simulink model "andbot1dot2_voltage_loop_frictioncompensation"  (R2015b)
settings: Solver=FixedStepAuto  StartTime=0.0  StopTime=simulation_time  FixedStep=0.04  RelTol=1e-3
values from neighbouring files (symbols this model uses):
  den_ff_Omega = [0 3.2393]    [andbot1dot2_MIMO_modeling_omega_loop.m]
  den_ff_Vel = [0 1.054]    [andbot1dot2_MIMO_modeling_vel_loop.m]
  den_Omega = [1 4.9887]    [andbot1dot2_MIMO_modeling.m]    (also in andbot1dot2_MIMO_modeling_omega_loop.m)
  den_Vel = [1 2.5006]    [andbot1dot2_MIMO_modeling.m]    (also in andbot1dot2_MIMO_modeling_vel_loop.m = [1 6.313])
  gain_anti_windup_Vel = 10    [andbot1dot2_MIMO_modeling_vel_loop.m]
  input_Omega = 1    [andbot1dot2_MIMO_modeling.m]
  input_Vel = 1    [andbot1dot2_MIMO_modeling.m]
  Ki_Omega = 0    [andbot1dot2_MIMO_modeling.m]    (also in andbot1dot2_MIMO_modeling_omega_loop.m = 5.8287)
  Ki_Vel = 1    [andbot1dot2_MIMO_modeling.m]    (also in andbot1dot2_MIMO_modeling_vel_loop.m = 21.3962)
  Kp_Omega = 1    [andbot1dot2_MIMO_modeling.m]    (also in andbot1dot2_MIMO_modeling_omega_loop.m = 4.4157)
  Kp_Vel = 1500    [andbot1dot2_MIMO_modeling.m]    (also in andbot1dot2_MIMO_modeling_vel_loop.m = 14.9624)
  num_ff_Omega = [0 4.99887]    [andbot1dot2_MIMO_modeling_omega_loop.m]
  num_ff_Vel = [0 6.313]    [andbot1dot2_MIMO_modeling_vel_loop.m]
  num_Omega = [0 3.2393]    [andbot1dot2_MIMO_modeling.m]    (also in andbot1dot2_MIMO_modeling_omega_loop.m)
  num_Vel = [0 0.261065]    [andbot1dot2_MIMO_modeling.m]    (also in andbot1dot2_MIMO_modeling_vel_loop.m = [0 1.054])
  Tsample = 0.04    [andbot1dot2_param.m]
  Vq_MAX = 1000    [andbot1dot2_param.m]
undefined symbols (not defined in the file or in its folder): ENCOutputMode, gain_anti_windup_Omega, PracLoopDelay, SetENCSample, Umax_Volt, Umin_Volt
libraries: cstblocks x4, realtime_pacer_lib x2, slctrlblks x1
settings Model: Creator=shangwei  LastModifiedBy=root

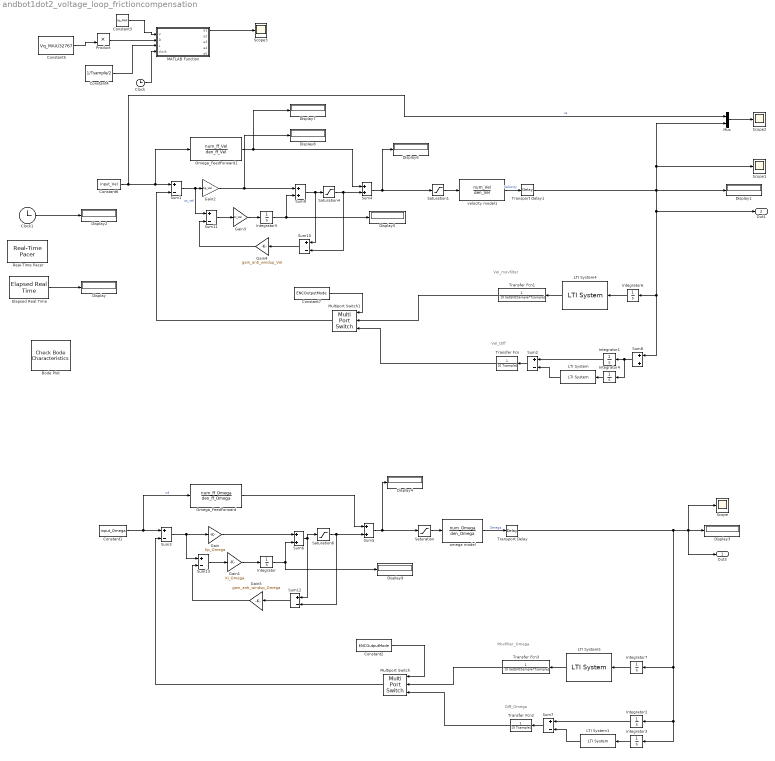
== system andbot1dot2_voltage_loop_frictioncompensation ==
  note: Vel_movfilter
  note: Diff_Omega
  note: Vel_Diff
  note: Movfilter_Omega
  Bode Plot : slctrlblks/Model Verification/Check Bode  Characteristics  InstantiateOnLoad=on  SaveOperatingPoints=off  LinearizationIOs={'/Sum1', 1, 'outin', 'on', '';'/Sum3', 1, 'outin', 'on', ''}  LinearizeAt=SnapshotTimes  SnapshotTimes=[0]  TriggerType=rising  SampleTime=auto  RateConversionMethod=zoh  PreWarpFreq=10  UseExactDelayModel=on  UseFullBlockNameLabels=off  UseBusSignalLabels=off  enabled=on  stopWhenAssertionFail=off  export=off  ViewDlgPos=[3023 418 520 393]  OpenViewOnLoad=off  LaunchViewOnOpen=on  FrequencyUnits=rad/s  MagnitudeUnits=dB  PhaseUnits=deg  TimeUnits=seconds  EnableUpperBound=off  UpperBoundFrequencies=[]  UpperBoundMagnitudes=[]  EnableLowerBound=off  LowerBoundFrequencies=[]  LowerBoundMagnitudes=[]
  Clock : Clock
  Clock1 : Clock
  Constant1 : Constant  Value=input_Omega  SampleTime=-1
  Constant2 : Constant  Value=ENCOutputMode  SampleTime=-1
  Constant3 : Constant  Value=Vq_MAX  SampleTime=-1
  Constant4 : Constant  Value=1/Tsample/2  SampleTime=-1
  Constant5 : Constant  Value=Vq_MAX/32767  SampleTime=-1
  Constant6 : Constant  Value=input_Vel  SampleTime=-1
  Constant7 : Constant  Value=ENCOutputMode  SampleTime=-1
  Display{,1..9} (10 alike) : Display
  Elapsed Real Time : realtime_pacer_lib/Elapsed Real Time
  Gain : Gain  Gain=Kp_Omega
  Gain1 : Gain  Gain=Ki_Omega
  Gain2 : Gain  Gain=Kp_Vel
  Gain3 : Gain  Gain=Ki_Vel
  Gain4 : Gain  Gain=gain_anti_windup_Vel
  Gain5 : Gain  Gain=gain_anti_windup_Omega
  Integrator{,1..7} (8 alike) : Integrator
  LTI System : cstblocks/LTI System  sys=time_delay_tf  IC=[]
  LTI System1 : cstblocks/LTI System  sys=time_delay_tf  IC=[]
  LTI System4 : cstblocks/LTI System  sys=(1 - exp(-SetENCSample*Tsample*tf('s'))) / (1 - exp(-Tsample*tf('s')))  IC=[]
  LTI System5 : cstblocks/LTI System  sys=(1 - exp(-SetENCSample*Tsample*tf('s'))) / (1 - exp(-Tsample*tf('s')))  IC=[]
  MATLAB Function : MATLAB Function  TreatAsAtomicUnit=on
  Multiport Switch : MultiPortSwitch  Inputs=2
  Multiport Switch1 : MultiPortSwitch  Inputs=2
  Mux : Mux  Inputs=2
  Omega_FeedForward : TransferFcn  Numerator=num_ff_Omega  Denominator=den_ff_Omega
  Omega_FeedForward1 : TransferFcn  Numerator=num_ff_Vel  Denominator=den_ff_Vel
  Product : Product
  Real-Time Pacer : realtime_pacer_lib/Real-Time Pacer  simTimePerRealTime=1
  Saturation{,1,4,6} (4 alike) : Saturate  UpperLimit=Umax_Volt  LowerLimit=Umin_Volt
  Scope{,1..3} (4 alike) : Scope
  Sum{1..3,7,10..13} (8 alike) : Sum  Inputs=+-
  Sum{4..6,8..9} (5 alike) : Sum
  Transfer Fcn : TransferFcn  Denominator=[0 Tsample]
  Transfer Fcn1 : TransferFcn  Denominator=[0 SetENCSample*Tsample]
  Transfer Fcn2 : TransferFcn  Denominator=[0 Tsample]
  Transfer Fcn3 : TransferFcn  Denominator=[0 SetENCSample*Tsample]
  Transport Delay : TransportDelay  DelayTime=PracLoopDelay
  Transport Delay1 : TransportDelay  DelayTime=PracLoopDelay
  omega model : TransferFcn  Numerator=num_Omega  Denominator=den_Omega
  velocity model1 : TransferFcn  Numerator=num_Vel  Denominator=den_Vel
  Out3 : Outport
  Out1 : Outport  Port=2
  wires:
  Sum3/1 -> Sum13/1, Gain/1
  Constant1/1 -> Sum3/1, Omega_FeedForward/1  "ud"
  Sum6/1 -> Saturation6/1, Sum12/1
  Sum1/1 -> Sum11/1, Gain2/1  "us_vel"
  velocity model1/1 -> Transport Delay1/1  "Velocity"
  Constant6/1 -> Mux/1, Sum1/1, Omega_FeedForward1/1  "us"
  omega model/1 -> Transport Delay/1  "Omega"
  Integrator3/1 -> LTI System1/1
  Integrator2/1 -> Sum7/1
  LTI System1/1 -> Sum7/2
  Sum7/1 -> Transfer Fcn2/1
  Sum2/1 -> Transfer Fcn/1
  Sum8/1 -> Integrator1/1, Integrator4/1
  Integrator1/1 -> Sum2/1
  LTI System/1 -> Sum2/2
  Integrator4/1 -> LTI System/1
  Constant3/1 -> MATLAB Function/1(V)
  MATLAB Function/1(a1) -> Scope3/1
  Product/1 -> MATLAB Function/2(D)
  Constant4/1 -> MATLAB Function/3(L)
  Clock/1 -> MATLAB Function/4(clock)
  Constant5/1 -> Product/2
  Multiport Switch/1 -> Sum3/2
  Transport Delay1/1 -> Display1/1, Scope1/1, Mux/2, Out1/1, Integrator6/1, Sum8/1
  Gain1/1 -> Integrator/1
  Gain/1 -> Sum6/1
  Elapsed Real Time/1 -> Display/1
  Clock1/1 -> Display2/1
  Multiport Switch1/1 -> Sum1/2
  Sum4/1 -> Display6/1, Saturation1/1
  Gain3/1 -> Integrator5/1
  Gain2/1 -> Display8/1, Sum9/1
  Sum9/1 -> Sum10/1, Saturation4/1
  Saturation/1 -> omega model/1
  Omega_FeedForward1/1 -> Display7/1, Sum4/1
  Mux/1 -> Scope2/1
  Saturation1/1 -> velocity model1/1
  Integrator/1 -> Sum6/2, Display9/1
  Integrator5/1 -> Sum9/2, Display5/1
  Omega_FeedForward/1 -> Sum5/1
  Saturation4/1 -> Sum4/2, Sum10/2
  Sum10/1 -> Gain4/1
  Gain4/1 -> Sum11/2
  Sum11/1 -> Gain3/1
  Sum5/1 -> Saturation/1, Display4/1
  Sum12/1 -> Gain5/1
  Saturation6/1 -> Sum12/2, Sum5/2
  Sum13/1 -> Gain1/1
  Gain5/1 -> Sum13/2
  Transport Delay/1 -> Integrator3/1, Integrator2/1, Integrator7/1, Scope/1, Out3/1, Display3/1
  Transfer Fcn2/1 -> Multiport Switch/3
  Constant2/1 -> Multiport Switch/1
  Transfer Fcn/1 -> Multiport Switch1/3
  Constant7/1 -> Multiport Switch1/1
  Integrator6/1 -> LTI System4/1
  LTI System4/1 -> Transfer Fcn1/1
  Integrator7/1 -> LTI System5/1
  LTI System5/1 -> Transfer Fcn3/1
  Transfer Fcn3/1 -> Multiport Switch/2
  Transfer Fcn1/1 -> Multiport Switch1/2

== matlab function andbot1dot2_voltage_loop_frictioncompensation/MATLAB Function ==
  data: V input; a1 output; D input; L input; a2 output; a3 output; a4 output; a5 output; clock input
function [a1,a2, a3, a4, a5]  = PWM_noise_sine(V, D, L, clock)
%#codegen
a = 1:5;

for n = 1:5
    a(n) = 2/ n * V / pi * sin(clock*pi*D);
end
a1 = a(1);
a2 = a(2);
a3 = a(3);
a4 = a(4);
a5 = a(5);
